simulink model "motorCC"  (R2018a)
settings: Solver=VariableStepAuto  StartTime=0.0  StopTime=100  RelTol=1e-3
settings Model: Creator=ttorea  LastModifiedBy=ttorea

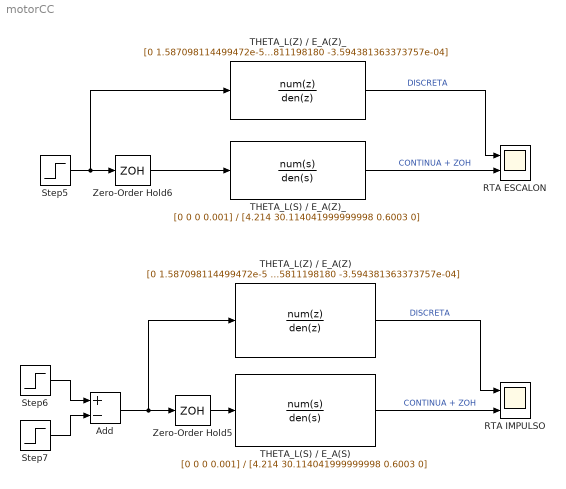
== system motorCC ==
  Add : Sum  Inputs=+-
  RTA ESCALON : Scope  NumInputPorts=2
  RTA IMPULSO : Scope  NumInputPorts=2
  Step5 : Step  Time=0  After=5  SampleTime=0
  Step6 : Step  Time=0  After=2  SampleTime=0
  Step7 : Step  Time=0.00001  After=2  SampleTime=0
  THETA_L(S) / E_A(S) : TransferFcn  Numerator=[0 0 0 0.001]  Denominator=[4.214 30.114041999999998 0.6003 0]
  THETA_L(S) / E_A(Z)_ : TransferFcn  Numerator=[0 0 0 0.001]  Denominator=[4.214 30.114041999999998 0.6003 0]
  THETA_L(Z) / E_A(Z) : DiscreteTransferFcn  Numerator=[0 1.587098114499472e-5 2.404465224969516e-5 6.336036425624988e-7]  Denominator=[1 -1.978426373061843 0.978785811198180 -3.594381363373757e-04]  SampleTime=1.1098
  THETA_L(Z) / E_A(Z)_ : DiscreteTransferFcn  Numerator=[0 1.587098114499472e-5 2.404465224969516e-5 6.336036425624988e-7]  Denominator=[1 -1.978426373061843 0.978785811198180 -3.594381363373757e-04]  SampleTime=1.1098
  Zero-Order Hold5 : ZeroOrderHold  SampleTime=1.1098
  Zero-Order Hold6 : ZeroOrderHold  SampleTime=1.1098
  wires:
  Step5/1 -> Zero-Order Hold6/1, THETA_L(Z) / E_A(Z)_/1
  THETA_L(Z) / E_A(Z)_/1 -> RTA ESCALON/1  "DISCRETA"
  Zero-Order Hold6/1 -> THETA_L(S) / E_A(Z)_/1
  THETA_L(S) / E_A(Z)_/1 -> RTA ESCALON/2  "CONTINUA + ZOH"
  THETA_L(Z) / E_A(Z)/1 -> RTA IMPULSO/1  "DISCRETA"
  Zero-Order Hold5/1 -> THETA_L(S) / E_A(S)/1
  THETA_L(S) / E_A(S)/1 -> RTA IMPULSO/2  "CONTINUA + ZOH"
  Step6/1 -> Add/1
  Step7/1 -> Add/2
  Add/1 -> THETA_L(Z) / E_A(Z)/1, Zero-Order Hold5/1
